simulink model "inductionmain"  (R2023b)
settings: Solver=ode3  StartTime=0.0  StopTime=1  FixedStep=0.0001  MaxStep=1e-4  RelTol=1e-3
libraries: spsVoltageMeasurementLib x3, spsAsynchronousMachineSIUnitsLib x1, fuzblock x1, spsGroundLib x1, spsPower3phInstantaneousLib x1, spsThreePhaseVIMeasurementLib x1, spsThreePhaseSourceLib x1, sps_lib x1
settings Model: Creator=malot  LastModifiedBy=DELL
settings DataIOCC: SaveFormat=Array  SignalLogging=off  DSMLogging=off  ReturnWorkspaceOutputs=off
settings RTWCC: GPUComputeCapability=5.0

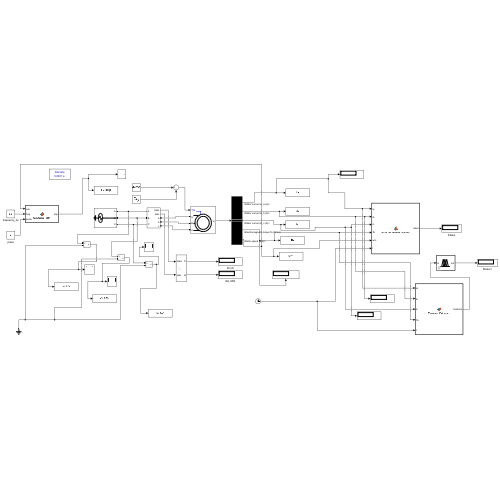
[thumbnail: Simulink's stored preview of the top-level diagram]
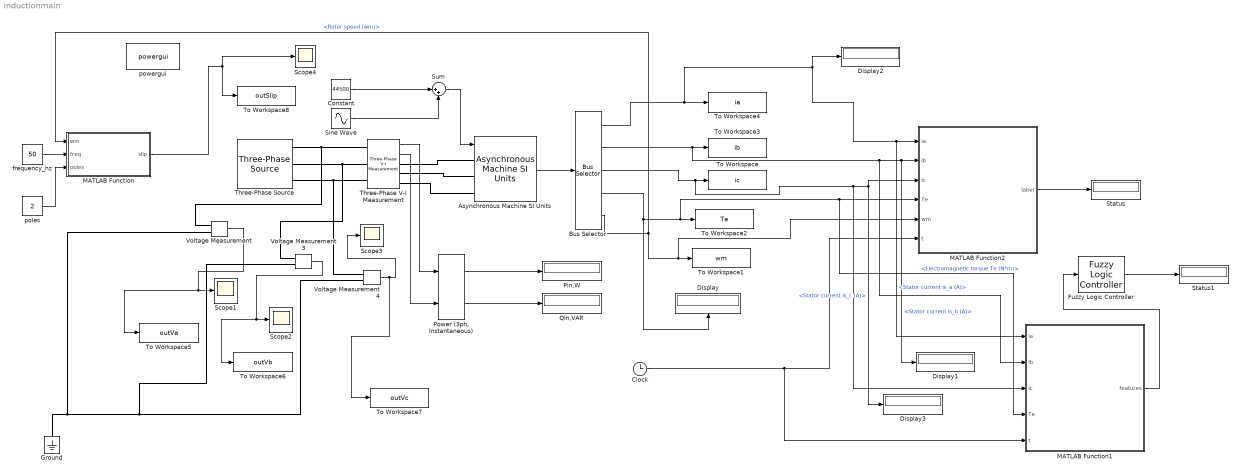
== system inductionmain ==
  Asynchronous Machine SI Units : spsAsynchronousMachineSIUnitsLib/Asynchronous Machine SI Units  RotorType=Squirrel-cage  PresetModel=No  MechanicalLoad=Torque Tm  ShowDetailedParameters=on  ReferenceFrame=Rotor  Units=SI  MeasurementBus=off  NominalParameters=[7000000 11000 50]  VoltageRatio=1  Stator=[0.732 0.048]  Rotor=[0.527 0.048]  Cage1=[0.433462 0.003960]  Cage2=[1671.921406 0.000000]  Lm=0.192  Mechanical=[2800 0.008 2]  PolePairs=2  InitialConditions=[0.01 0 0 0 0 0 0 0]  SimulateSaturation=off  Saturation=[14.03593122, 27.81365428, 53.79336849, 72.68890987, 97.98006896, 148.6815601, 215.7428561, 302.9841135, 428.7778367 ; 230, 322, 414, 460, 506, 552, 598, 644, 690]  LoadFlowParameters=1492000  TsPowergui=0  TsBlock=-1  IterativeModel=Trapezoidal non iterative  IterativeDiscreteModel=Trapezoidal non iterative  Pmec=1.492e+006
  Bus Selector : BusSelector  OutputSignals=Stator measurements.Stator current is_a (A),Stator measurements.Stator current is_b (A),Stator measurements.Stator current is_c (A),Mechanical.Electromagnetic torque Te (N*m),Mechanical.Rotor speed (wm)
  Clock : Clock
  Constant : Constant  Value=44500
  Display{,1..3} (4 alike) : Display
  Fuzzy Logic Controller : fuzblock/Fuzzy Logic  Controller  FIS=fis  OutputSampleNumber=101  DataType=double  FuzzifiedInputs=off  RuleFiringStrengths=off  RuleOutputs=off  AggregatedOutputs=off  SimulateUsing=Interpreted execution  OutOfRangeInputValueMessage=warning  NoRuleFiredMessage=warning  EmptyOutputFuzzySetMessage=warning
  Ground : spsGroundLib/Ground  LConnTagsString=a
  MATLAB Function : MATLAB Function  TreatAsAtomicUnit=on
  MATLAB Function1 : MATLAB Function  TreatAsAtomicUnit=on
  MATLAB Function2 : MATLAB Function  TreatAsAtomicUnit=on
  Pin,W : Display
  "Power (3ph, Instantaneous)" : spsPower3phInstantaneousLib/Power (3ph, Instantaneous)
  Qin,VAR : Display
  Scope{1..4} (4 alike) : Scope
  Sine Wave : Sin  Amplitude=0  Frequency=20  SampleTime=0
  Status : Display
  Status1 : Display
  Sum : Sum  Inputs=|++
  Three-Phase V-I Measurement : spsThreePhaseVIMeasurementLib/Three-Phase V-I Measurement  VoltageMeasurement=phase-to-ground  SetLabelV=off  LabelV=Vabc  Vpu=off  VpuLL=off  CurrentMeasurement=yes  SetLabelI=off  LabelI=Iabc  Ipu=off  Pbase=100e6  Vbase=500e3  OutputType=Complex  PhasorSimulation=off  PSBequivalent=0
  Three-Phase Source : spsThreePhaseSourceLib/Three-Phase Source  InternalConnection=Yg  VoltagePhases=on  Voltage=[6256.25496285992 6256.25496285992 6256.25496285992]  PhaseAngle=0  Voltage_phases=[6350.85,6350.85,6350.85]  PhaseAngles_phases=[0 -120 +120]  Frequency=50  NonIdealSource=off  SpecifyImpedance=off  Resistance=0.8929  Inductance=16.58e-3  ShortCircuitLevel=100e6  BaseVoltage=25e3  XRratio=7  BusType=swing  Pref=10e3  Qref=0  Prefabc=[10e3, 10e3, 10e3]  Qrefabc=[0, 0, 0]  Qmin=-inf  Qmax=inf
  To Workspace : ToWorkspace  VariableName=ic  SampleTime=-1
  To Workspace1 : ToWorkspace  VariableName=wm  SampleTime=-1
  To Workspace2 : ToWorkspace  VariableName=Te  SampleTime=-1
  To Workspace3 : ToWorkspace  VariableName=ib  SampleTime=-1
  To Workspace4 : ToWorkspace  VariableName=ia  SampleTime=-1
  To Workspace5 : ToWorkspace  VariableName=outVa  SaveFormat=Timeseries  SampleTime=-1
  To Workspace6 : ToWorkspace  VariableName=outVb  SaveFormat=Timeseries  SampleTime=-1
  To Workspace7 : ToWorkspace  VariableName=outVc  SaveFormat=Timeseries  SampleTime=-1
  To Workspace8 : ToWorkspace  VariableName=outSlip  SampleTime=-1
  Voltage Measurement : spsVoltageMeasurementLib/Voltage Measurement  PhasorSimulation=off  OutputType=Complex  PSBequivalent=0
  Voltage Measurement3 : spsVoltageMeasurementLib/Voltage Measurement  PhasorSimulation=off  OutputType=Complex  PSBequivalent=0
  Voltage Measurement4 : spsVoltageMeasurementLib/Voltage Measurement  PhasorSimulation=off  OutputType=Complex  PSBequivalent=0
  frequency_hz : Constant  Value=50
  poles : Constant  Value=2
  powergui : sps_lib/powergui  Priority=1  SimulationMode=Discrete  SampleTime=1e-4  frequency=60  Iterations=50  frequencyindice=50  Pbase=100e6  ErrMax=1e-4  UnitsV=kV  UnitsW=MW  buscounter=0  FunctionMessages=off  echomessages=off  EnableUseOfTLC=off  CurrentSourceSwitches=off  DisableSnubberDevices=off  DisableRonSwitches=off  DisableVfSwitches=off  DisplayEquations=off  AutomaticDiscreteSolvers=off  SolverType=Tustin/Backward Euler (TBE)  Interpol=off  ExternalGateDelay=off  methode=off  Ts=100  x0status=blocks  SPID=on  SwTol=0  HookPort=off  NonlinearTolerance=1e-4  nMaxIteration=100  ContinueOnMaxIteration=off  RestoreLinks=warning  ResistiveCurrentMeasurement=off  Frange=[0:2:500]  Ylog=off  Xlog=on  ShowGrid=off  save=off  variable=ZData  structure=0  ZoomFFT=off  StartTime=0.0  cycles=1  DisplayStyle=1  fundamental=60  FreqAxis=off  MaxFrequency=1000  frequencyindicesteady=1  RmsSteady=1  display=off
  wires:
  Three-Phase V-I Measurement/1 -> "Power (3ph, Instantaneous)"/1
  Three-Phase V-I Measurement/2 -> "Power (3ph, Instantaneous)"/2
  "Power (3ph, Instantaneous)"/1 -> Pin,W/1
  "Power (3ph, Instantaneous)"/2 -> Qin,VAR/1
  Asynchronous Machine SI Units/1 -> Bus Selector/1
  Bus Selector/3 -> MATLAB Function1/3(ic), Display3/1, MATLAB Function2/3(ic), To Workspace/1  "<Stator current is_c (A)>"
  Bus Selector/5 -> MATLAB Function/1(wm), MATLAB Function2/5(wm), To Workspace1/1  "<Rotor speed (wm)>"
  Bus Selector/4 -> MATLAB Function1/4(Te), MATLAB Function2/4(Te), To Workspace2/1, Display/1  "<Electromagnetic torque Te (N*m)>"
  Bus Selector/2 -> MATLAB Function1/2(ib), Display1/1, MATLAB Function2/2(ib), To Workspace3/1  "<Stator current is_b (A)>"
  Bus Selector/1 -> MATLAB Function1/1(ia), MATLAB Function2/1(ia), Display2/1, To Workspace4/1  "<Stator current is_a (A)>"
  Voltage Measurement/1 -> Scope1/1, To Workspace5/1
  Voltage Measurement3/1 -> To Workspace6/1, Scope2/1
  Voltage Measurement4/1 -> To Workspace7/1, Scope3/1
  frequency_hz/1 -> MATLAB Function/2(freq)
  poles/1 -> MATLAB Function/3(poles)
  MATLAB Function/1(slip) -> Scope4/1, To Workspace8/1
  MATLAB Function2/1(label) -> Status/1
  Clock/1 -> MATLAB Function1/5(t), MATLAB Function2/6(t)
  Constant/1 -> Sum/1
  Sine Wave/1 -> Sum/2
  Sum/1 -> Asynchronous Machine SI Units/1
  MATLAB Function1/1(features) -> Fuzzy Logic Controller/1
  Fuzzy Logic Controller/1 -> Status1/1
  connections:
  Three-Phase Source/RConn1 -- Three-Phase V-I Measurement/LConn1 -- Voltage Measurement/LConn1
  Three-Phase Source/RConn2 -- Voltage Measurement3/LConn1 -- Three-Phase V-I Measurement/LConn2
  Three-Phase Source/RConn3 -- Voltage Measurement4/LConn1 -- Three-Phase V-I Measurement/LConn3
  Three-Phase V-I Measurement/RConn3 -- Asynchronous Machine SI Units/LConn3
  Three-Phase V-I Measurement/RConn2 -- Asynchronous Machine SI Units/LConn2
  Three-Phase V-I Measurement/RConn1 -- Asynchronous Machine SI Units/LConn1
  Voltage Measurement/LConn2 -- Voltage Measurement4/LConn2 -- Voltage Measurement3/LConn2 -- Ground/LConn1

== matlab function inductionmain/MATLAB Function1 ==
  data: ia input; ib input; ic input; features output double size=1; Te input; t input
function features = Feature_Extractor(ia, ib, ic, Te, t)

%#codegen
features = zeros(1,4);   % VERY IMPORTANT

persistent Te_avg learned baseline_Te

if isempty(Te_avg)
    Te_avg = 0;
    baseline_Te = 0;
    learned = 0;
end

% Filter currents (simple smoothing)
alpha = 0.01;
ia = alpha*abs(ia) + (1-alpha)*abs(ia);
ib = alpha*abs(ib) + (1-alpha)*abs(ib);
ic = alpha*abs(ic) + (1-alpha)*abs(ic);

% Average current
I_avg = (ia + ib + ic) / 3;

if I_avg < 1e-3
    features = [0 100 100 0];
    return;
end

% -------------------------
% Learn baseline torque
% -------------------------
if t < 1.5
    baseline_Te = baseline_Te + abs(Te);
    learned = learned + 1;
    features = [0 100 100 0];
    return;
end

if learned > 0 && learned < 99999
    baseline_Te = baseline_Te / learned;
    learned = 99999;
end

% -------------------------
% Feature Calculation
% -------------------------

% Current imbalance
I_max = max([ia ib ic]);
I_min = min([ia ib ic]);
current_imbalance = ((I_max - I_min) / I_avg) * 100;

% Torque level (auto-normalized)
if baseline_Te > 0
    torque_level = (abs(Te) / baseline_Te) * 100;
else
    torque_level = 100;
end

% Min phase current
min_phase_current = (I_min / I_avg) * 100;

% Torque ripple
Te_avg = 0.99*Te_avg + 0.01*Te;
torque_ripple = (abs(Te - Te_avg) / (abs(Te_avg)+1)) * 100;

features(1) = current_imbalance;
features(2) = torque_level;
features(3) = min_phase_current;
features(4) = torque_ripple;

== matlab function inductionmain/MATLAB Function ==
  data: wm input; slip output; freq input; poles input
function slip = calculate_slip(wm, freq, poles)
    % Calculate slip for induction motor
    % Inputs:
    %   wm    - Rotor speed (rad/s)
    %   freq  - Supply frequency (Hz)
    %   poles - Number of poles
    % Output:
    %   slip  - Slip (per unit, 0 to 1)

    % Calculate synchronous speed in RPM
    n_sync = (120 * freq) / poles;

    % Convert rotor speed from rad/s to RPM
    n_actual = wm * 60 / (2 * pi);

    % Calculate slip
    slip = (n_sync - n_actual) / n_sync;

    % Ensure slip is bounded (safety check)
    if slip < 0
        slip = 0;
    elseif slip > 1
        slip = 1;
    end
end

== matlab function inductionmain/MATLAB Function2 ==
  data: ia input; ib input; ic input; label output double size=1; Te input; wm input; t input
function label = ThresholdFaultClassifier(ia, ib, ic, Te, wm, t)

    % --- 1. SETUP PERSISTENT VARIABLES ---
    persistent Ia_filt Ib_filt Ic_filt Te_avg
    if isempty(Ia_filt)
        Ia_filt = 0; Ib_filt = 0; Ic_filt = 0; Te_avg = 0;
    end

    % --- 2. CURRENT FILTER (Keep this as is) ---
    alpha_I = 0.001; 
    Ia_filt = (1 - alpha_I) * Ia_filt + alpha_I * abs(ia);
    Ib_filt = (1 - alpha_I) * Ib_filt + alpha_I * abs(ib);
    Ic_filt = (1 - alpha_I) * Ic_filt + alpha_I * abs(ic);
    
    % --- 3. TORQUE FILTER (THE CRITICAL FIX) ---
    % Changed alpha from 0.05 to 0.0001
    % This makes the filter extremely slow, so it captures the "DC Average".
    % Now, when Te vibrates, Te_avg will stay flat, creating a large difference.
    alpha_T = 0.0001; 
    Te_avg = (1 - alpha_T) * Te_avg + alpha_T * Te;

    % --- 4. IGNORE STARTUP ---
    if t < 0.5
        label = 0;
        return;
    end

    % --- 5. CALCULATE METRICS ---
    I_avg = (Ia_filt + Ib_filt + Ic_filt) / 3;
    if I_avg < 1, label = 0; return; end

    max_dev = max([abs(Ia_filt - I_avg), abs(Ib_filt - I_avg), abs(Ic_filt - I_avg)]);
    imb_ratio = max_dev / I_avg;

    % Torque Ripple Calculation
    % Now (Te - Te_avg) will be large because Te_avg is "frozen"
    torque_ripple = abs(Te - Te_avg) / (abs(Te_avg) + 1);

    % --- 6. CLASSIFICATION ---
    
    if imb_ratio > 0.40 
        label = 3; % Stator Fault

    elseif torque_ripple > 0.15 
        label = 2; % Broken Rotor Bar (This should now trigger!)

    elseif imb_ratio > 0.04 
        label = 1; % Voltage Unbalance

    else
        label = 0; % Healthy
    end

end
